simulink model "mpcsimulink2019"  (R2019b)
settings: Solver=VariableStepAuto  StartTime=0.0  StopTime=20  RelTol=1e-3
values from neighbouring files (symbols this model uses):
  d = 1    [INIT.m]    (also in INITKF.m; INITexp.m; INITnonmpc.m; pendcont.m)
  D = 0    [INIT.m]    (also in INITexp.m; pendcont.m = m*L*L*(M+m*(1-Cy^2)))
  g = -10    [INIT.m]    (also in INITKF.m; INITexp.m = -9.8; INITnonmpc.m = -9.8; pendcont.m = -9.8)
  K = lqr(A,B,Q,R)    [INIT.m]    (also in INITKF.m; INITexp.m; INITnonmpc.m)
  L = 2    [INIT.m]    (also in INITKF.m; INITexp.m = 0.07; INITnonmpc.m = 0.06; pendcont.m = 0.06)
  M = 5    [INIT.m]    (also in INITKF.m; INITexp.m = 0.32; INITnonmpc.m = 0.08; pendcont.m = 0.08)
  m = 1    [INIT.m]    (also in INITKF.m; INITexp.m = 0.25; INITnonmpc.m = 0.01; pendcont.m = 0.01)
  Ts = 0.1    [INITnonmpc.m]
  y0 = [0;0;0.1;0]    [INITexp.m]
libraries: mpclib x1
settings Model: Creator=Prodigio  LastModifiedBy=Prodigio
settings DataIOCC: ReturnWorkspaceOutputs=off
settings DebuggingCC: ArithmeticOperatorsInVariantConditions=warning
settings SFSimCC: SimUseLocalCustomCode=off  CustomCodeUndefinedFunction=UseInterfaceOnly
settings RTWCC: RTWUseLocalCustomCode=off

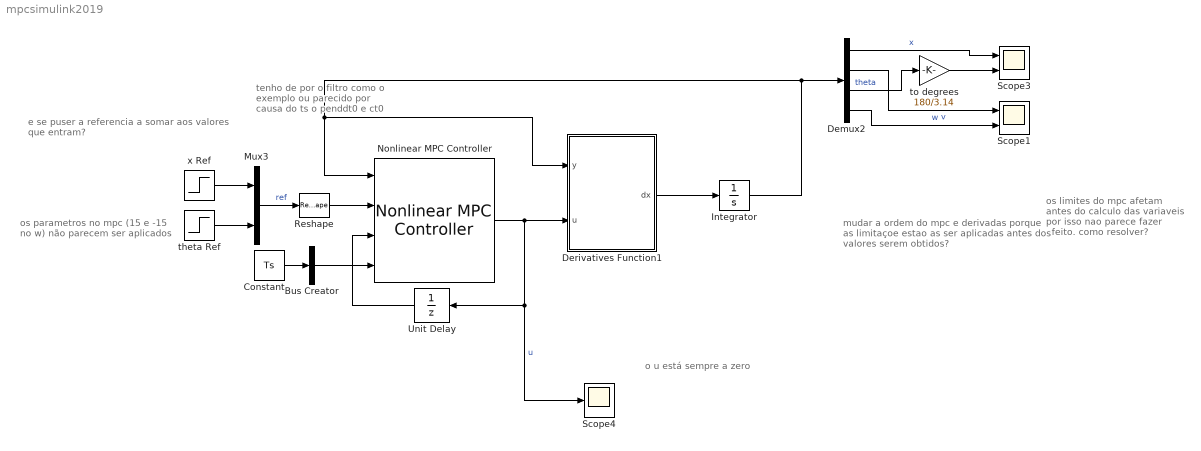
== system mpcsimulink2019 ==
  note: tenho de por o filtro como o exemplo ou parecido por causa do ts o penddt0 e ct0
  note: os limites do mpc afetam antes do calculo das variaveis por isso nao parece fazer efeito.
      | como resolver?
  note: mudar a ordem do mpc e derivadas porque as limitaçoe estao as ser aplicadas antes dos valores serem obtidos?
  note: e se puser a referencia a somar aos valores que entram?
  note: os parametros no mpc (15 e -15 no w) não parecem ser aplicados
  note: o u está sempre a zero
  Bus Creator : BusCreator  Inputs=1  OutDataTypeStr=Bus: BusNMPC  NonVirtualBus=on
      settings: InheritFromInputs=off
  Constant : Constant  Value=Ts
  Demux2 : Demux
  Derivatives Function1 : MATLAB Function  TreatAsAtomicUnit=on
  Integrator : Integrator  InitialCondition=[0;y0(2);pi;y0(4)]
  Mux3 : Mux  Inputs=2
  Nonlinear MPC Controller : mpclib/Nonlinear MPC Controller  SCDEnableBlockLinearizationSpecification=on  nlmpcobj=nlobj  UseObjectTs=on  UseMEX=off  md_enabled=off  mvtarget_enabled=off  param_enabled=on  cost_enabled=off  mvseq_enabled=off  stateseq_enabled=off  ovseq_enabled=off  slack_enabled=off  status_enabled=off  ov_min=off  ov_max=off  mv_min=off  mv_max=off  mvrate_min=off  mvrate_max=off  state_min=off  state_max=off  ov_weight=off  mv_weight=off  mvrate_weight=off  ecr_weight=off  nlp_initialize=off
  Reshape : Reshape  OutputDimensionality=Row vector (2-D)
  Scope1 : Scope  NumInputPorts=2
  Scope3 : Scope  NumInputPorts=2
  Scope4 : Scope
  Unit Delay : UnitDelay  SampleTime=-1  HasFrameUpgradeWarning=on
  theta Ref : Step  Time=11  After=0  SampleTime=0
  to degrees : Gain  Gain=180/3.14
  x Ref : Step  Time=7  After=0.2  SampleTime=0
  wires:
  Demux2/1 -> Scope3/1  "x"
  Nonlinear MPC Controller/1 -> Scope4/1, Unit Delay/1, Derivatives Function1/2(u)  "u"
  Derivatives Function1/1(dx) -> Integrator/1
  theta Ref/1 -> Mux3/2
  x Ref/1 -> Mux3/1
  Constant/1 -> Bus Creator/1
  Bus Creator/1 -> Nonlinear MPC Controller/4
  Reshape/1 -> Nonlinear MPC Controller/2
  Mux3/1 -> Reshape/1  "ref"
  Demux2/2 -> Scope1/1  "v"
  Demux2/4 -> Scope1/2  "w"
  Integrator/1 -> Nonlinear MPC Controller/1, Derivatives Function1/1(y), Demux2/1
  Unit Delay/1 -> Nonlinear MPC Controller/3
  to degrees/1 -> Scope3/2
  Demux2/3 -> to degrees/1  "theta"

== matlab function mpcsimulink2019/Derivatives Function1 ==
  settings: updateMethod=CONTINUOUS
  data: y input; dx output; m parameter; M parameter; L parameter; g parameter; d parameter; K parameter; u input
function dx = derivativesexp(y,m, M, L, g, d, K,u)
% y = [x , ^x, o , ^o] states , y=xdot
% M massa do carro, m massa do pendulo, L tamanho do fio
% d fricÃ§ao, g grav no pendulo

dx=0*y;
Sy = sin(y(3));
Cy = cos(y(3));
D = m*L*L*(M+m*(1-Cy^2));

% setpoints
% newx = [2; 0; pi; 0];
% newx = [0; 0; 0; 0];
% 
% % if(t>12)
% %     newx = [-1; 0; pi; 0]; 
% % end 
% 
% % open loop (no control)
% % if(t>29)
% %   u = 0;
% % else
%                                             % && u ~= 0
% if (( y(3) > (pi-pi/5) ) && ( y(3) < (pi+pi/5)) || ...
%    ( y(3) > (-pi-pi/5) ) && ( y(3) < (-pi+pi/5)) )  
%     u = K * ([0;0;pi;0] - [y(1);y(2);y(3);y(4)]); % lqr control u = k*(newx-x)
% else
%     % energy based swing-up control % 1996 furata and astrom eq.6
%     % E=2/3*m2*l^2*x(4)^2 - m2*g*l*(cos(x(3))-1);
%     % u=0.2*m1*E*x(4)*cos(x(3));
% %         k=1;
% %         Ed= -m*g*L*cos(pi);
% %         E= m*L^2*y(4) - m*g*L*cos(y(3));
% %         u=k*y(4)*(E-Ed);
%      E= m*g*L*(cos(y(3)));
%      u=0.8*M*E*y(4)*(cos(y(3))); %velocidade com que ganha balanço, 0.8 ou o primeiro valor serve como tunning
% %     end
% end



%derivadas 

dx(1,1) = y(2);
dx(2,1) = (1/D)*(-m^2*L^2*g*Cy*Sy + m*L^2*(m*L*y(4)^2*Sy - d*y(2))) + m*L*L*(1/D)*u;
dx(3,1) = y(4);
dx(4,1) = (1/D)*((m+M)*m*g*L*Sy - m*L*Cy*(m*L*y(4)^2*Sy - d*y(2))) - m*L*Cy*(1/D)*u;


% -m*m*l*l*g*Sy*Sy
% m*l*l*m*l*y(4)^2*Sy
% %-m*l*l*d*y(2)
% %m*l*l*u
% 
% (m+M)*m*g*l*Sy
% m*l*Cy*m*l*y(4)^2*Sy
% %-m*l*Cy*d*y(2)
% %m*l*Cy*u
